simulink model "Exercitiul1"  (R2016a)
settings: Solver=VariableStepDiscrete  StartTime=0.0  StopTime=10.0  RelTol=1e-3
undefined symbols (not defined in the file): m
settings Model: Creator=Cristina  LastModifiedBy=Cristina

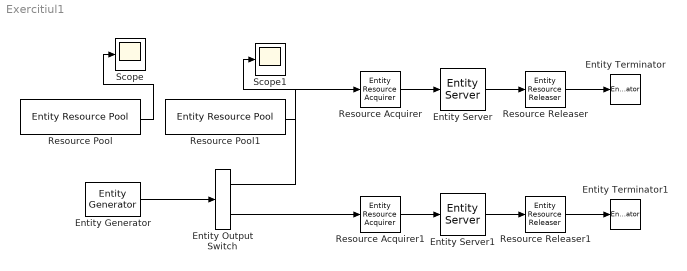
== system Exercitiul1 ==
  Entity Output Switch : EntityOutputSwitch  InputPortMessageModes=m  OutputPortMessageModes=m,m  SwitchingCriterion=From attribute  SwitchAttributeName=Type
  Entity Generator : EntityGenerator  OutputPortMessageModes=m  TimeSource=MATLAB action  IntergenerationTimeAction=dt = 0.01 + 0.19 * rand;  GenerateAction=|  AttributeName=Type|ServiceTime  AttributeInitialValue=0|1  EntityType=Structured  EntityTypeName=Entity
      | if rand < 0.4
      |     entity.Type = 1;
      |     entity.ServiceTime = 0.5
      | else
      |     entity.Type = 2;
      |     entity.ServiceTime = 0.7;
  Entity Server : EntityServer  InputPortMessageModes=m  OutputPortMessageModes=m  Capacity=4  ServiceTimeSource=Attribute  ServiceTimeValue=0.5
  Entity Server1 : EntityServer  InputPortMessageModes=m  OutputPortMessageModes=m  Capacity=8  ServiceTimeSource=Attribute  ServiceTimeValue=0.7
  Entity Terminator : EntityTerminator  InputPortMessageModes=m
  Entity Terminator1 : EntityTerminator  InputPortMessageModes=m
  Resource Acquirer : EntityResourceAcquirer  InputPortMessageModes=m  OutputPortMessageModes=m  NumberWaitingEntities=6  ResourceName=ResourceType1
      settings: OutputPortMap=o3
  Resource Acquirer1 : EntityResourceAcquirer  InputPortMessageModes=m  OutputPortMessageModes=m  NumberWaitingEntities=10  ResourceName=ResourceType2
      settings: OutputPortMap=o3
  Resource Releaser : EntityResourceReleaser  InputPortMessageModes=m  OutputPortMessageModes=m  ResourceToRelease=Selected  ResourceName=ResourceType1
  Resource Releaser1 : EntityResourceReleaser  InputPortMessageModes=m  OutputPortMessageModes=m  ResourceToRelease=Selected  ResourceName=ResourceType2
  Resource Pool : EntityResourcePool  ResourceName=ResourceType1  ResourceAmount=4  AmountInUse=on
  Resource Pool1 : EntityResourcePool  ResourceName=ResourceType2  ResourceAmount=8  AmountInUse=on
  Scope : Scope
  Scope1 : Scope
  wires:
  Entity Generator/1 -> Entity Output Switch/1
  Entity Output Switch/1 -> Resource Acquirer/1
  Entity Output Switch/2 -> Resource Acquirer1/1
  Resource Acquirer1/1 -> Entity Server1/1
  Resource Acquirer/1 -> Entity Server/1
  Entity Server/1 -> Resource Releaser/1
  Entity Server1/1 -> Resource Releaser1/1
  Resource Releaser/1 -> Entity Terminator/1
  Resource Releaser1/1 -> Entity Terminator1/1
  Resource Pool/1 -> Scope/1
  Resource Pool1/1 -> Scope1/1
